simulink model "adcs_v16_integral_light_sun_sgp_igrf_power_7May2012"  (Simulink 7.5)
settings: Solver=ode1  StartTime=0.0  StopTime=120000  FixedStep=s_SIM_STEP_SIZE  RelTol=1e-3
values from neighbouring files (symbols this model uses):
  A = ((T_SIDE + .29)*1e-3)^2    [constants_v13.m]    (also in constants_v15.m; constants_v15_Pow.m; constants_v15_Pow_ss_error.m; constants_v16_integral_kartavya.m)
  Area_SP_S1 = 4*11*0.02025*0.04025    (= 0.03586275)    [constants_v15_Pow.m]    (also in constants_v15_Pow_ss_error.m; constants_v16_integral_light_sun_sgp_igrf_power_13Dec2011.m)
  Area_SP_S2 = 4*11*0.02025*0.04025    (= 0.03586275)    [constants_v15_Pow.m]    (also in constants_v15_Pow_ss_error.m; constants_v16_integral_light_sun_sgp_igrf_power_13Dec2011.m)
  Area_SP_S3 = 0.0    (= 0)    [constants_v15_Pow.m]    (also in constants_v15_Pow_ss_error.m; constants_v16_integral_light_sun_sgp_igrf_power_13Dec2011.m)
  Area_SP_S4 = 4*11*0.02025*0.04025    (= 0.03586275)    [constants_v15_Pow.m]    (also in constants_v15_Pow_ss_error.m; constants_v16_integral_light_sun_sgp_igrf_power_13Dec2011.m)
  Area_SP_S5 = 0.0    (= 0)    [constants_v15_Pow.m]    (also in constants_v15_Pow_ss_error.m; constants_v16_integral_light_sun_sgp_igrf_power_13Dec2011.m)
  Area_SP_S6 = 3*11*0.02025*0.04025    (= 0.0268970625)    [constants_v15_Pow.m]    (also in constants_v15_Pow_ss_error.m; constants_v16_integral_light_sun_sgp_igrf_power_13Dec2011.m)
  Ca_Solar_Drag = 1.4    [constants_v13.m]    (also in constants_v15.m; constants_v15_Pow.m; constants_v15_Pow_ss_error.m; constants_v16_integral_kartavya.m)
  Cd = 2.2    [constants_v13.m]    (also in constants_v15.m; constants_v15_Pow.m; constants_v15_Pow_ss_error.m; constants_v16_integral_kartavya.m)
  check_time = 60000    [constants_v13.m]    (also in constants_v15.m = 10000; constants_v15_Pow.m = 10000; constants_v15_Pow_ss_error.m = 10000; constants_v16_integral_kartavya.m = 10000)
  efficiany_solar_cell = 0.16    [constants_v15_Pow.m]    (also in constants_v15_Pow_ss_error.m; constants_v16_integral_light_sun_sgp_igrf_power_13Dec2011.m)
  equinox = datenum('21-Mar-2010 12:0:0')    [constants_v13.m]    (also in constants_v15.m; constants_v15_Pow.m; constants_v15_Pow_ss_error.m; constants_v16_integral_kartavya.m)
  I_MAX = 0.5    [constants_v13.m]    (also in constants_v15.m; constants_v15_Pow.m; constants_v15_Pow_ss_error.m; constants_v16_integral_kartavya.m)
  I_TORQUER = 3.6 / 7.31    (= 0.492476060192)    [constants_v13.m]    (also in constants_v15.m; constants_v15_Pow.m; constants_v15_Pow_ss_error.m; constants_v16_integral_kartavya.m)
  Kd = 2* m_INERTIA / (s_numOrbits * T_ORBIT )    [constants_v13.m]    (also in constants_v15.m = m_INERTIA * (2 + delta)* zeta * w; constants_v15_Pow.m = m_INERTIA * (2 + delta)* zeta * w; constants_v15_Pow_ss_error.m = m_INERTIA * (2 + delta)* zeta * w; constants_v16_integral_kartavya.m = m_INERTIA * (2 + delta)* zeta * w)
  Kdetumb = K_det*eye(3)    [constants_v13.m]    (also in constants_v15.m; constants_v15_Pow.m; constants_v15_Pow_ss_error.m; constants_v16_integral_kartavya.m)
  Ki = m_INERTIA * delta * zeta * w^3    [constants_v15.m]    (also in constants_v15_Pow.m; constants_v15_Pow_ss_error.m; constants_v16_integral_kartavya.m; constants_v16_integral_light_sun_sgp_igrf_power_13Dec2011.m)
  Kp = m_INERTIA / (s_numOrbits * T_ORBIT * zeta)^2    [constants_v13.m]    (also in constants_v15.m = m_INERTIA * (w*w + 2*delta*zeta^2*w^2); constants_v15_Pow.m = m_INERTIA * (w*w + 2*delta*zeta^2*w^2); constants_v15_Pow_ss_error.m = m_INERTIA * (w*w + 2*delta*zeta^2*w^2); constants_v16_integral_kartavya.m = m_INERTIA * (w*w + 2*delta*zeta^2*w^2))
  m_INERTIA = [Ixx Ixy Ixz; Ixy Iyy Iyz; Ixz Iyz Izz]    [constants_v13.m]    (also in constants_v15.m; constants_v15_Pow.m = 1*[Ixx Ixy Ixz; Ixy Iyy Iyz; Ixz Iyz Izz]; constants_v15_Pow_ss_error.m = 1*[Ixx Ixy Ixz; Ixy Iyy Iyz; Ixz Iyz Izz]; constants_v16_integral_kartavya.m)
  mu = 6.673e-11*5.9742e24    (= 398658366000000)    [constants_v13.m]    (also in constants_v15.m; constants_v15_Pow.m; constants_v15_Pow_ss_error.m; constants_v16_integral_kartavya.m)
  N = 40    [constants_v13.m]    (also in constants_v15.m; constants_v15_Pow.m; constants_v15_Pow_ss_error.m; constants_v16_integral_kartavya.m)
  P_momentum_flux_from_the_sun = 4.4e-6    (= 4.4e-06)    [constants_v13.m]    (also in constants_v15.m; constants_v15_Pow.m; constants_v15_Pow_ss_error.m; constants_v16_integral_kartavya.m)
  q_BI0 = euler2qBI(roll0,pitch0,yaw0)    [constants_v13.m]    (also in constants_v15.m; constants_v15_Pow.m; constants_v15_Pow_ss_error.m; constants_v16_integral_kartavya.m)
  s_FRAME_SIZE = 2    [constants_v13.m]    (also in constants_v15.m; constants_v15_Pow.m; constants_v15_Pow_ss_error.m; constants_v16_integral_kartavya.m)
  s_m_MAX = 0.95    [constants_v13.m]    (also in constants_v15.m; constants_v15_Pow.m; constants_v15_Pow_ss_error.m; constants_v16_integral_kartavya.m)
  s_MAG_B = 2.5e-5    (= 2.5e-05)    [constants_v13.m]    (also in constants_v15.m; constants_v15_Pow.m; constants_v15_Pow_ss_error.m; constants_v16_integral_kartavya.m)
  s_MAGMETER_WEIGHT = .9    (= 0.9)    [constants_v13.m]    (also in constants_v15.m; constants_v15_Pow.m; constants_v15_Pow_ss_error.m; constants_v16_integral_kartavya.m)
  s_SIM_STEP_SIZE = 0.1    [constants_v13.m]    (also in constants_v15.m; constants_v15_Pow.m; constants_v15_Pow_ss_error.m; constants_v16_integral_kartavya.m)
  s_SS_ADC_gain = 5    [constants_v13.m]    (also in constants_v15.m; constants_v15_Pow.m; constants_v15_Pow_ss_error.m; constants_v16_integral_kartavya.m)
  s_SS_ADC_res = 2^12 - 1    (= 4095)    [constants_v13.m]    (also in constants_v15.m; constants_v15_Pow.m; constants_v15_Pow_ss_error.m; constants_v16_integral_kartavya.m)
  s_SS_MAX_ANGLE = 85    [constants_v13.m]    (also in constants_v15.m; constants_v15_Pow.m; constants_v15_Pow_ss_error.m; constants_v16_integral_kartavya.m)
  s_TAU_W = 60    [constants_v13.m]    (also in constants_v15.m; constants_v15_Pow.m; constants_v15_Pow_ss_error.m; constants_v16_integral_kartavya.m)
  s_x_MAGMETER_BIAS = 50e-9    (= 5e-08)    [constants_v13.m]    (also in constants_v15.m; constants_v15_Pow.m; constants_v15_Pow_ss_error.m; constants_v16_integral_kartavya.m)
  side = 0.26    [constants_v13.m]    (also in constants_v15.m; constants_v15_Pow.m; constants_v15_Pow_ss_error.m; constants_v16_integral_kartavya.m)
  Snum = 6    [constants_v13.m]    (also in constants_v15.m; constants_v15_Pow.m; constants_v15_Pow_ss_error.m; constants_v16_integral_kartavya.m)
  Solar_Constant = 1353    [constants_v15_Pow.m]    (also in constants_v15_Pow_ss_error.m; constants_v16_integral_light_sun_sgp_igrf_power_13Dec2011.m)
  today = datenum('18-Oct-2010 10:30:0')    [constants_v13.m]    (also in constants_v15.m; constants_v15_Pow.m; constants_v15_Pow_ss_error.m; constants_v16_integral_kartavya.m)
  tol_q4 = 0.7    [constants_v13.m]    (also in constants_v15.m = 0.85; constants_v15_Pow.m = 0.85; constants_v15_Pow_ss_error.m = 0.85; constants_v16_integral_kartavya.m = 0.85)
  tol_w = 4e-3    (= 0.004)    [constants_v13.m]    (also in constants_v15.m; constants_v15_Pow.m; constants_v15_Pow_ss_error.m; constants_v16_integral_kartavya.m)
  tolw_n2d = 10e-3    (= 0.01)    [constants_v15.m]    (also in constants_v15_Pow.m; constants_v15_Pow_ss_error.m; constants_v16_integral_kartavya.m; constants_v16_integral_light_sun_sgp_igrf_power_13Dec2011.m)
  Ts_display = 6    [constants_v13.m]    (also in constants_v15.m; constants_v15_Pow.m; constants_v15_Pow_ss_error.m; constants_v16_integral_kartavya.m)
  v_COM_to_COP_b = [.2; 1.75; .2]*1e-2    [constants_v13.m]    (also in constants_v15.m; constants_v15_Pow.m; constants_v15_Pow_ss_error.m; constants_v16_integral_kartavya.m)
  v_S1 = [1 0 0]    [constants_v13.m]    (also in constants_v15.m; constants_v15_Pow.m; constants_v15_Pow_ss_error.m; constants_v16_integral_kartavya.m)
  v_S2 = [-1 0 0]    [constants_v13.m]    (also in constants_v15.m; constants_v15_Pow.m; constants_v15_Pow_ss_error.m; constants_v16_integral_kartavya.m)
  v_S3 = [0 1 0]    [constants_v13.m]    (also in constants_v15.m; constants_v15_Pow.m; constants_v15_Pow_ss_error.m; constants_v16_integral_kartavya.m)
  v_S4 = [0 -1 0]    [constants_v13.m]    (also in constants_v15.m; constants_v15_Pow.m; constants_v15_Pow_ss_error.m; constants_v16_integral_kartavya.m)
  v_S5 = [0 0 1]    [constants_v13.m]    (also in constants_v15.m; constants_v15_Pow.m; constants_v15_Pow_ss_error.m; constants_v16_integral_kartavya.m)
  v_S6 = [0 0 -1]    [constants_v13.m]    (also in constants_v15.m; constants_v15_Pow.m; constants_v15_Pow_ss_error.m; constants_v16_integral_kartavya.m)
  v_x_MOUNTING_THETA_ZYX_BODY_TORQUER = [1; 1; 1]* pi/180    [constants_v13.m]    (also in constants_v15.m; constants_v15_Pow.m; constants_v15_Pow_ss_error.m; constants_v16_integral_kartavya.m)
  wx0 = 2*pi/180    (= 0.0349065850399)    [constants_v13.m]    (also in constants_v15.m = 0.00174532925199; constants_v15_Pow.m = 1.74532925199e-05; constants_v15_Pow_ss_error.m = 2.01533262693e-05; constants_v16_integral_kartavya.m = 0.0174532925199)
  wy0 = 1*pi/180    (= 0.0174532925199)    [constants_v13.m]    (also in constants_v15.m = 0.00174532925199; constants_v15_Pow.m = 1.74532925199e-05; constants_v15_Pow_ss_error.m = 2.01533262693e-05; constants_v16_integral_kartavya.m = 0)
  wz0 = -2*pi/180    (= -0.0349065850399)    [constants_v13.m]    (also in constants_v15.m = 0.00174532925199; constants_v15_Pow.m = 1.74532925199e-05; constants_v15_Pow_ss_error.m = 2.01533262693e-05; constants_v16_integral_kartavya.m = -0.00872664625997)
libraries: simulink x9, commnoisgen2 x7, aerolibutil x2
(part 2 of 2)

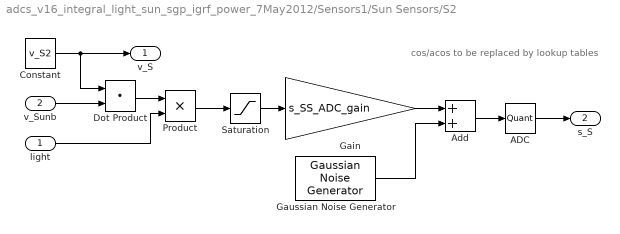
== system adcs_v16_integral_light_sun_sgp_igrf_power_7May2012/Sensors1/Sun Sensors/S2 ==
  note: cos/acos to be replaced by lookup tables
  light : Inport  OutDataType=sfix(16)  OutScaling=2^0
  v_Sunb : Inport  Port=2  OutDataType=sfix(16)  OutScaling=2^0
  ADC : Quantizer  QuantizationInterval=1/s_SS_ADC_res
  Add : Sum  OutDataType=sfix(16)  OutScaling=2^-10
  Constant : Constant  Value=v_S2  OutDataType=sfix(16)  OutScaling=2^0
  Dot Product : DotProduct  OutDataType=sfix(16)  OutScaling=2^-10  InputSameDT=on  OutDataTypeStr=Inherit: Inherit via internal rule
  Gain : Gain  Gain=s_SS_ADC_gain  ParameterDataType=sfix(16)  ParameterScaling=2^0  OutDataType=sfix(16)  OutScaling=2^0
  Gaussian Noise Generator : commnoisgen2/Gaussian Noise Generator  SystemSampleTime=-1  m=0  d=s_x_SUNSENSOR  s=41  Ts=s_SIM_STEP_SIZE  frameBased=off  sampPerFrame=1  orient=off  outDataType=double
  Product : Product  OutDataType=fixdt(1, 16)  OutScaling=2^0  RndMeth=Zero
  Saturation : Saturate  UpperLimit=inf  LowerLimit=0  OutDataType=sfix(16)  OutScaling=2^0
  v_S : Outport  OutDataType=sfix(16)  OutScaling=2^0
  s_S : Outport  Port=2  OutDataType=sfix(16)  OutScaling=2^0
  wires:
  ADC/1 -> s_S/1
  Add/1 -> ADC/1
  Gain/1 -> Add/1
  Gaussian Noise Generator/1 -> Add/2
  Constant/1 -> Dot Product/1, v_S/1
  Saturation/1 -> Gain/1
  v_Sunb/1 -> Dot Product/2
  Dot Product/1 -> Product/1
  Product/1 -> Saturation/1
  light/1 -> Product/2

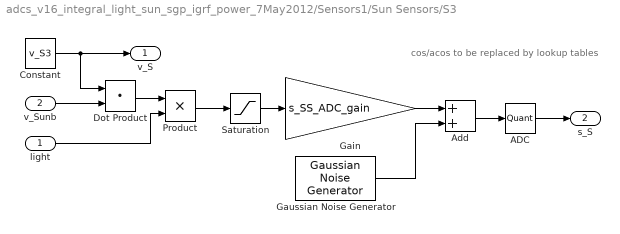
== system adcs_v16_integral_light_sun_sgp_igrf_power_7May2012/Sensors1/Sun Sensors/S3 ==
  note: cos/acos to be replaced by lookup tables
  light : Inport  OutDataType=sfix(16)  OutScaling=2^0
  v_Sunb : Inport  Port=2  OutDataType=sfix(16)  OutScaling=2^0
  ADC : Quantizer  QuantizationInterval=1/s_SS_ADC_res
  Add : Sum  OutDataType=sfix(16)  OutScaling=2^-10
  Constant : Constant  Value=v_S3  OutDataType=sfix(16)  OutScaling=2^0
  Dot Product : DotProduct  OutDataType=sfix(16)  OutScaling=2^-10  InputSameDT=on  OutDataTypeStr=Inherit: Inherit via internal rule
  Gain : Gain  Gain=s_SS_ADC_gain  ParameterDataType=sfix(16)  ParameterScaling=2^0  OutDataType=sfix(16)  OutScaling=2^0
  Gaussian Noise Generator : commnoisgen2/Gaussian Noise Generator  SystemSampleTime=-1  m=0  d=s_x_SUNSENSOR  s=41  Ts=s_SIM_STEP_SIZE  frameBased=off  sampPerFrame=1  orient=off  outDataType=double
  Product : Product  OutDataType=fixdt(1, 16)  OutScaling=2^0  RndMeth=Zero
  Saturation : Saturate  UpperLimit=inf  LowerLimit=0  OutDataType=sfix(16)  OutScaling=2^0
  v_S : Outport  OutDataType=sfix(16)  OutScaling=2^0
  s_S : Outport  Port=2  OutDataType=sfix(16)  OutScaling=2^0
  wires:
  light/1 -> Product/2
  Product/1 -> Saturation/1
  Dot Product/1 -> Product/1
  v_Sunb/1 -> Dot Product/2
  Saturation/1 -> Gain/1
  Constant/1 -> v_S/1, Dot Product/1
  Gaussian Noise Generator/1 -> Add/2
  Gain/1 -> Add/1
  Add/1 -> ADC/1
  ADC/1 -> s_S/1

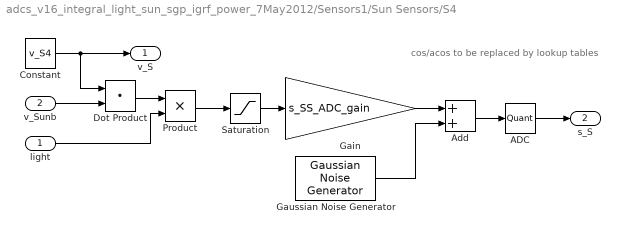
== system adcs_v16_integral_light_sun_sgp_igrf_power_7May2012/Sensors1/Sun Sensors/S4 ==
  note: cos/acos to be replaced by lookup tables
  light : Inport  OutDataType=sfix(16)  OutScaling=2^0
  v_Sunb : Inport  Port=2  OutDataType=sfix(16)  OutScaling=2^0
  ADC : Quantizer  QuantizationInterval=1/s_SS_ADC_res
  Add : Sum  OutDataType=sfix(16)  OutScaling=2^-10
  Constant : Constant  Value=v_S4  OutDataType=sfix(16)  OutScaling=2^0
  Dot Product : DotProduct  OutDataType=sfix(16)  OutScaling=2^-10  InputSameDT=on  OutDataTypeStr=Inherit: Inherit via internal rule
  Gain : Gain  Gain=s_SS_ADC_gain  ParameterDataType=sfix(16)  ParameterScaling=2^0  OutDataType=sfix(16)  OutScaling=2^0
  Gaussian Noise Generator : commnoisgen2/Gaussian Noise Generator  SystemSampleTime=-1  m=0  d=s_x_SUNSENSOR  s=41  Ts=s_SIM_STEP_SIZE  frameBased=off  sampPerFrame=1  orient=off  outDataType=double
  Product : Product  OutDataType=fixdt(1, 16)  OutScaling=2^0  RndMeth=Zero
  Saturation : Saturate  UpperLimit=inf  LowerLimit=0  OutDataType=sfix(16)  OutScaling=2^0
  v_S : Outport  OutDataType=sfix(16)  OutScaling=2^0
  s_S : Outport  Port=2  OutDataType=sfix(16)  OutScaling=2^0
  wires:
  ADC/1 -> s_S/1
  Add/1 -> ADC/1
  Gain/1 -> Add/1
  Gaussian Noise Generator/1 -> Add/2
  Constant/1 -> Dot Product/1, v_S/1
  Saturation/1 -> Gain/1
  v_Sunb/1 -> Dot Product/2
  Dot Product/1 -> Product/1
  Product/1 -> Saturation/1
  light/1 -> Product/2

== system adcs_v16_integral_light_sun_sgp_igrf_power_7May2012/Sensors1/Sun Sensors/S5 ==
  note: cos/acos to be replaced by lookup tables
  light : Inport  OutDataType=sfix(16)  OutScaling=2^0
  v_Sunb : Inport  Port=2  OutDataType=sfix(16)  OutScaling=2^0
  ADC : Quantizer  QuantizationInterval=1/s_SS_ADC_res
  Add : Sum  OutDataType=sfix(16)  OutScaling=2^-10
  Constant : Constant  Value=v_S5  OutDataType=sfix(16)  OutScaling=2^0
  Dot Product : DotProduct  OutDataType=sfix(16)  OutScaling=2^-10  InputSameDT=on  OutDataTypeStr=Inherit: Inherit via internal rule
  Gain : Gain  Gain=s_SS_ADC_gain  ParameterDataType=sfix(16)  ParameterScaling=2^0  OutDataType=sfix(16)  OutScaling=2^0
  Gaussian Noise Generator : commnoisgen2/Gaussian Noise Generator  SystemSampleTime=-1  m=0  d=s_x_SUNSENSOR  s=41  Ts=s_SIM_STEP_SIZE  frameBased=off  sampPerFrame=1  orient=off  outDataType=double
  Product : Product  OutDataType=fixdt(1, 16)  OutScaling=2^0  RndMeth=Zero
  Saturation : Saturate  UpperLimit=inf  LowerLimit=0  OutDataType=sfix(16)  OutScaling=2^0
  v_S : Outport  OutDataType=sfix(16)  OutScaling=2^0
  s_S : Outport  Port=2  OutDataType=sfix(16)  OutScaling=2^0
  wires:
  light/1 -> Product/2
  Product/1 -> Saturation/1
  Dot Product/1 -> Product/1
  v_Sunb/1 -> Dot Product/2
  Saturation/1 -> Gain/1
  Constant/1 -> v_S/1, Dot Product/1
  Gaussian Noise Generator/1 -> Add/2
  Gain/1 -> Add/1
  Add/1 -> ADC/1
  ADC/1 -> s_S/1

== system adcs_v16_integral_light_sun_sgp_igrf_power_7May2012/Sensors1/Sun Sensors/S6 ==
  note: cos/acos to be replaced by lookup tables
  light : Inport  OutDataType=sfix(16)  OutScaling=2^0
  v_Sunb : Inport  Port=2  OutDataType=sfix(16)  OutScaling=2^0
  ADC : Quantizer  QuantizationInterval=1/s_SS_ADC_res
  Add : Sum  OutDataType=sfix(16)  OutScaling=2^-10
  Constant : Constant  Value=v_S6  OutDataType=sfix(16)  OutScaling=2^0
  Dot Product : DotProduct  OutDataType=sfix(16)  OutScaling=2^-10  InputSameDT=on  OutDataTypeStr=Inherit: Inherit via internal rule
  Gain : Gain  Gain=s_SS_ADC_gain  ParameterDataType=sfix(16)  ParameterScaling=2^0  OutDataType=sfix(16)  OutScaling=2^0
  Gaussian Noise Generator : commnoisgen2/Gaussian Noise Generator  SystemSampleTime=-1  m=0  d=s_x_SUNSENSOR  s=41  Ts=s_SIM_STEP_SIZE  frameBased=off  sampPerFrame=1  orient=off  outDataType=double
  Product : Product  OutDataType=fixdt(1, 16)  OutScaling=2^0  RndMeth=Zero
  Saturation : Saturate  UpperLimit=inf  LowerLimit=0  OutDataType=sfix(16)  OutScaling=2^0
  v_S : Outport  OutDataType=sfix(16)  OutScaling=2^0
  s_S : Outport  Port=2  OutDataType=sfix(16)  OutScaling=2^0
  wires:
  ADC/1 -> s_S/1
  Add/1 -> ADC/1
  Gain/1 -> Add/1
  Gaussian Noise Generator/1 -> Add/2
  Constant/1 -> Dot Product/1, v_S/1
  Saturation/1 -> Gain/1
  v_Sunb/1 -> Dot Product/2
  Dot Product/1 -> Product/1
  Product/1 -> Saturation/1
  light/1 -> Product/2

== matlab function Torquer/Embedded MATLAB Function4 ==
  data: euler input double; DCM output double
function DCM  = f(euler)
% This block supports the Embedded MATLAB subset.
% See the help menu for details. 

roll = euler(1);
pitch = euler(2);
yaw = euler(3);

rot_x = [  1         0           0;...
             0         cos(roll)  sin(roll);...
             0        -sin(roll)  cos(roll)];
         
rot_y = [cos(pitch)   0       -sin(pitch);...
            0           1        0;...
           sin(pitch)   0        cos(pitch)];
       
rot_z = [ cos(yaw) sin(yaw) 0;...
           -sin(yaw) cos(yaw) 0;...
            0        0            1];
         
DCM  = rot_z *  rot_y *  rot_x;

== matlab function Embedded MATLAB Function ==
  data: x input double; u input double; xdot output double; m_INERTIA parameter double
function xdot = fcn(x, u, m_INERTIA)
% This block supports the Embedded MATLAB subset.
% See the help menu for details. 

q = x(1:4);
w = x(5:7);

W = ...
    [ 0 w(3) -w(2) w(1);
      -w(3) 0 w(1) w(2);
      w(2) -w(1) 0 w(3);
      -w(1) -w(2) -w(3) 0];
  
  qdot = 0.5 * W * q;
  wdot = inv(m_INERTIA)*( u - cross( w, m_INERTIA*w ) );
  
  xdot = [qdot; wdot];

== matlab function I -> B/L_Inertial ==
  data: x input double; v_B output double; v_I input double
function v_B = fcn(x, v_I)
% This block supports the Embedded MATLAB subset.
% See the help menu for details. 

q = x(1:4);

q0 = q(4); q1 = q(1); q2 = q(2); q3 = q(3);

TBI = [ q0^2 + q1^2 - q2^2 - q3^2,         2*q0*q3 + 2*q1*q2,         2*q1*q3 - 2*q0*q2;
           2*q1*q2 - 2*q0*q3, q0^2 - q1^2 + q2^2 - q3^2,         2*q0*q1 + 2*q2*q3;
           2*q0*q2 + 2*q1*q3,         2*q2*q3 - 2*q0*q1, q0^2 - q1^2 - q2^2 + q3^2];

v_B =  TBI*v_I;

== matlab function q -> w/Subsystem6/(1-L) + L/z ==
  data: a input double; y output double; b input double
function y = fcn(a,b)
%#eml

c = 1-a;

y = c+b;
if y>1
    y=1;
end

== matlab function q-normalise ==
  data: x input double; xN output double
function xN  = fcn(x)
% This block gives DCM for converting from ECI to ORBIT frames
% inputs: state vector in ECI
% output: DCM

q = x(1:4);
q = q/sqrt(dot(q,q));
xN = [q; x(5:7)];

== matlab function External Torques/Subsystem/Solar_drag ==
  data: v_Sun_b input double; solar_drag output double; Ca_Solar_Drag parameter double; P_momentum_flux_from_the_sun parameter double; light input double; side parameter double
function solar_drag = fcn(v_Sun_b,Ca_Solar_Drag,P_momentum_flux_from_the_sun,light, side)
% This block supports the Embedded MATLAB subset.
% See the help menu for details. 

% dot product of area vector and sun vector
if (norm(v_Sun_b) == 0)
    u = [1;0;0];
else
    u = v_Sun_b / norm(v_Sun_b);
end

y = 0 ;
a = side;
a = a*a; %Area of satellite
b =  zeros(3,6);
b(:,1) = a*[1;0;0];
b(:,2) = a*[0;1;0];
b(:,3) = a*[0;0;1];
b(:,4) = a*[-1;0;0];
b(:,5) = a*[0;-1;0];
b(:,6) = a*[0;0;-1];

x = 0;
for i=1:6
     x = dot(b(:,i),u);
    if(x>0)
            y = y+x;
    end
end
Ap = y;

solar_drag = -Ap * Ca_Solar_Drag * P_momentum_flux_from_the_sun * u * light;

== matlab function External Torques/L_Inertial ==
  data: x input double; tau output double; v_Si input double; mu parameter double; m_INERTIA parameter double
function tau = fcn(x, v_Si, mu, m_INERTIA)
% This block supports the Embedded MATLAB subset.
% See the help menu for details. 

q = x(1:4);

q0 = q(4); q1 = q(1); q2 = q(2); q3 = q(3);

TBI = [ q0^2 + q1^2 - q2^2 - q3^2,         2*q0*q3 + 2*q1*q2,         2*q1*q3 - 2*q0*q2;
           2*q1*q2 - 2*q0*q3, q0^2 - q1^2 + q2^2 - q3^2,         2*q0*q1 + 2*q2*q3;
           2*q0*q2 + 2*q1*q3,         2*q2*q3 - 2*q0*q1, q0^2 - q1^2 - q2^2 + q3^2];

r_I = v_Si(1:3);
r_B =  TBI*r_I;

R = sqrt(dot(r_B, r_B));
tau = 3*mu * cross( r_B, m_INERTIA*r_B) / R^5;

== matlab function Control Law/q->w ==
  data: B output double; B_l input double; B_k input double; dB output double; s_FRAME_SIZE parameter double
function [B, dB] = fcn(B_l, B_k, s_FRAME_SIZE)
% This block supports the Embedded MATLAB subset.
% See the help menu for details. 

dB = (B_l - B_k)/s_FRAME_SIZE;
B = (B_l + B_k)/2;

== matlab function QuEST ==
  data: v_Bb_m input double; m_SUN input double; q_BO_est output double; v_Bo_c input double; v_So_c input double; s_SS_ADC_gain parameter double; Snum parameter double; light_est output double; s_MAGMETER_WEIGHT parameter double; s_SS_MAX_ANGLE parameter double; v_Sun1 output double
function [q_BO_est, light_est, v_Sun1] = QuEST(v_Bb_m,m_SUN,v_Bo_c,v_So_c, s_SS_ADC_gain, Snum, s_MAGMETER_WEIGHT, s_SS_MAX_ANGLE)

    % Help
    % q_triad = Estimated quaternion
    % b1,b2 = the 2 measurement vectors in body frames
    % r1,r2 = the 2 measurement vectors in reference frames (orbit/inertial; orbit used)
    % b1 is the measurement with very high accurace as compared to b2
    % I am not sure how r1 and r2 will be determined
    % a1 and a2 are Relative weights of b1 and b2


%%%%% calculate v_Sb_m from m_SUN %%%%
t_S = ones(1,Snum)*cos(s_SS_MAX_ANGLE *pi/180);
m_SUN(4,:) = 1.0*(m_SUN(5,:)>t_S);     % set flags from measured voltages

values = m_SUN(5,:);

n_SS = 0;
for i=1:Snum
    if values(i) < 0.5*s_SS_ADC_gain
        n_SS = n_SS + 1;
    end
end

if (n_SS == Snum) 
    light = 0;
else
    light = 1;
end

light_est = light;
%v_Sun1 = [1;0;0];

if (light == 1)    
    
    %%% CALCULATE SUN VECTOR %%%
    
    ssvectors = zeros(3); ssvalues = zeros(3,1); ssflags = zeros(3,1);
     % flags = m_SUN(4,:)';
%     for i=1:3
%         [~, index] = sort(m_SUN(5,:));  % sort values in ascending order
%         z = index(Snum);
%         ssvectors(i,1:3) = m_SUN(1:3,z)';
%         ssflags(i) = m_SUN(4,z);
%         ssvalues(i) = m_SUN(5,z);
%         m_SUN(5,z) = -100 ;
%         for j= 1:Snum
%             if( norm(ssvectors(i,1:3)+m_SUN(1:3,j)') == 0 )
%                 m_SUN(5,j) = -100;
%             end
%         end
%     end
    
    [~, index] = sort(m_SUN(5,:));  % sort values in ascending order
    z = index(Snum); p = 0; % first vector
    ssvectors(1,1:3) = m_SUN(1:3,z)';
    ssvalues(1) = m_SUN(5,z);
    p = p+1;
    
    z = index(Snum-p);  % second vector
    while norm(m_SUN(1:3,z)' + ssvectors(1,1:3)) == 0
        p = p+1;
        z = index(Snum - p);
    end
    ssvectors(2,1:3) = m_SUN(1:3,z)';
    ssvalues(2) = m_SUN(5,z);
    p = p+1;
    
    z = index(Snum-p);  % 3rd vector
    while (norm(m_SUN(1:3,z)' + ssvectors(1,1:3)) == 0) || (norm(m_SUN(1:3,z)' + ssvectors(2,1:3)) == 0)
        p = p+1;
        z = index(Snum - p);
    end
    ssvectors(3,1:3) = m_SUN(1:3,z)';
    ssvalues(3) = m_SUN(5,z);
%     p = p+1;
    
    % v_Sun1 = inv(ssvectors)*ssvalues;
    v_Sun1 = ssvectors\ssvalues;
    v_Sun1 = v_Sun1/sqrt(dot(v_Sun1, v_Sun1));
    v_Sb_m = v_Sun1/sqrt(dot(v_Sun1, v_Sun1));
    
    %%%% start TRIAD %%%%

    b1 = v_Bb_m;
    b2 = v_Sb_m;
    r1 = v_Bo_c;
    r2 = v_So_c;

    a1 = s_MAGMETER_WEIGHT;
    a2 = 1-a1;

    %b3
    b3 = cross(b1,b2);
    b3 = b3/norm(b3) ;
    %r3
    r3 = cross(r1,r2);
    r3 = r3/norm(r3) ;

    %mu
    mu = ( 1 + dot(b3,r3) ) * ( a1*dot(b1,r1) + a2*dot(b2,r2) ) ;
    mu =  mu + dot( cross(b3,r3) , ( a1*cross(b1,r1) + a2*cross(b2,r2) ) ) ;

    %nu
    nu = dot( ( b3 + r3 ) , ( a1*cross(b1,r1) + a2*cross(b2,r2) )  ) ;

    %rho
    rho = sqrt( mu*mu + nu*nu );

    %q
    if( mu > 0)
        k_q_triad = (1/( 2*sqrt( rho*(rho+mu)*( 1 + dot(b3,r3) ) ) ) );
        v_q_triad = ( rho + mu )*( cross(b3,r3) ) + nu*(b3 + r3) ;
        s_q_triad = ( rho + mu )* ( 1 + dot(b3,r3) ) ;
        q_triad = [v_q_triad ; s_q_triad];
        q_triad = k_q_triad * q_triad ;
    else
        k_q_triad = (1/( 2*sqrt( rho*(rho-mu)*( 1 + dot(b3,r3) ) ) ) );
        v_q_triad = ( nu )*( cross(b3,r3) ) + ( rho - mu )*(b3 + r3) ;
        s_q_triad = ( nu )* ( 1 + dot(b3,r3) ) ;
        q_triad = [v_q_triad ; s_q_triad];
        q_triad = k_q_triad * q_triad ;    
    end

    q_triad = q_triad / sqrt(dot(q_triad,q_triad)) ;
    q_BO_est = q_triad;
else
    v_Sun1 = [1 ; 0 ; 0];
    q_BO_est = [0;0;0;1];
    flag_sum = 0;
end
end

== matlab function Satellite Computations I Propagators/m_TOI_NEW1 ==
  data: v_I input double; ECI input double; v_O output double
function v_O  = fcn(v_I, ECI)
% This block gives DCM for converting from ECI to ORBIT frames
% inputs: state vector in ECI
% output: DCM

r = ECI(1:3);   % position vector in ECI
v = ECI(4:6);   % velocity vector in ECI

oy = cross(v,r);    % orbit frame x...
oy = oy/sqrt(dot(oy,oy));

oz = -r/sqrt(dot(r,r));

ox = cross(oy,oz);
ox = ox/sqrt(dot(ox,ox));

TOI = [ox oy oz]';

v_O = TOI*v_I;

== matlab function Control Law/Nominal ==
  data: ieu output double; ieu_prev input double; eu output double; m output double; light input double; w input double; m_N output double; v_B input double; Kp parameter double; Kd parameter double; Ki parameter double; q input double; s_FRAME_SIZE parameter double
function [ieu, eu, m, m_N] = fcn(ieu_prev, light, w, v_B, Kp, Kd, Ki, q, s_FRAME_SIZE)
% This block supports the Embedded MATLAB subset.
% See the help menu for details. 

Bnorm = sqrt(dot(v_B, v_B));

q = q/sqrt(dot(q,q));

qv = q(1:3);    % e*sin(t/2)
qs = q(4);      %   cos(t/2)

eu = 2*qv*qs;     % 2*e*sin(t/2)*cos(t/2) = e*sin(t)    % P variable
         
ieu = ieu_prev + eu*s_FRAME_SIZE;   % integral eu dt,   % I variable

m = (Kp*eu + Ki*ieu + Kd*w) / Bnorm^2;

m_N = cross( m, v_B ) * light;

== matlab function Subsystem1/f: I->B ==
  data: x input double; v_B output double; v_I input double
function v_B = fcn(x, v_I)
% This block supports the Embedded MATLAB subset.
% See the help menu for details. 

q = x(1:4);

q0 = q(4); q1 = q(1); q2 = q(2); q3 = q(3);

TBI = [ q0^2 + q1^2 - q2^2 - q3^2,         2*q0*q3 + 2*q1*q2,         2*q1*q3 - 2*q0*q2;
           2*q1*q2 - 2*q0*q3, q0^2 - q1^2 + q2^2 - q3^2,         2*q0*q1 + 2*q2*q3;
           2*q0*q2 + 2*q1*q3,         2*q2*q3 - 2*q0*q1, q0^2 - q1^2 - q2^2 + q3^2];

v_B =  TBI*v_I;
v_B = v_B/sqrt(dot(v_B,v_B));

== matlab function External Torques/Aerodynamic Torque/aero torque ==
  data: v_B input double; u_aero output double; side parameter double; Cd parameter double; v_COM_to_COP_b parameter double
function u_aero = fcn( v_B,side, Cd, v_COM_to_COP_b)

% x = 1;
% z = x*1;
% y = z*u;

% This block supports an embeddable subset of the MATLAB language.
% See the help menu for details. 
% dot product of area vector and velocity vector
rho   = 1e-10;
vnorm = sqrt(dot(v_B,v_B));
v_unit = v_B / vnorm;

y = 0 ;
a = side;
a = a*a; %Area of satellite
b =  zeros(3,6);
b(:,1) = a*[1;0;0];
b(:,2) = a*[0;1;0];
b(:,3) = a*[0;0;1];
b(:,4) = a*[-1;0;0];
b(:,5) = a*[0;-1;0];
b(:,6) = a*[0;0;-1];

for i=1:6
     x = dot(b(:,i),v_unit);
    if(x>0)
            y = y+x;
    end
end
Ap = y; % total exposed area

F_aero = -0.5 * Cd * rho * Ap * vnorm^2 * v_unit;

u_aero = cross(v_COM_to_COP_b, F_aero);

== matlab function Power D0D/Watts x time/Embedded MATLAB Function ==
  data: Latitude input double; Longitude input double; Downlink_power output double; flag_downlink output double; flag_france output double; flag_india output double
function [Downlink_power, flag_downlink,flag_france,flag_india]  = fcn(Latitude, Longitude)
%#eml
phi = 10;
flag_france = 0;
flag_india = 0;
if (Latitude - 22.5833)^2 + cos(Latitude*pi/180)*(Longitude - 82.7666)^2 < (15 + phi)^2
    flag_downlink = 1;
    flag_india = 1;
elseif (Latitude - 48.8)^2 + cos(Latitude*pi/180)*(Longitude - 2.33)^2 < phi^2
    flag_downlink = 1;
    flag_france = 1;
else
    flag_downlink = 0;
end

Downlink_power = flag_downlink*2.6; %W
    
% 
% y = u;

== matlab function External Torques/Aerodynamic Torque/v_I to v_B ==
  data: v_I input double; x input double; v_B output double
function v_B = fcn(v_I,x)
% This block supports the Embedded MATLAB subset.
% See the help menu for details. 

q = x(1:4);

q0 = q(4); q1 = q(1); q2 = q(2); q3 = q(3);

TBI = [ q0^2 + q1^2 - q2^2 - q3^2,         2*q0*q3 + 2*q1*q2,         2*q1*q3 - 2*q0*q2;
           2*q1*q2 - 2*q0*q3, q0^2 - q1^2 + q2^2 - q3^2,         2*q0*q1 + 2*q2*q3;
           2*q0*q2 + 2*q1*q3,         2*q2*q3 - 2*q0*q1, q0^2 - q1^2 - q2^2 + q3^2];

v_B =  TBI*v_I;

== matlab function Sensors1/Sun Sensors/Embedded MATLAB Function ==
  data: v_S1 input double; m_SUN output double; s_S1 input double; v_S2 input double; s_S2 input double; v_S3 input double; s_S3 input double; v_S4 input double; s_S4 input double; v_S5 input double; s_S5 input double; v_S6 input double; s_S6 input double; Snum parameter double; s_SS_MAX_ANGLE parameter double; values output double
function [m_SUN, values] = fcn(v_S1, s_S1, v_S2, s_S2, v_S3, s_S3, v_S4, s_S4, v_S5, s_S5, v_S6, s_S6, Snum, s_SS_MAX_ANGLE)

a = cos(s_SS_MAX_ANGLE *pi/180);
t_S = ones(1,6)*a;

m_SUNtot = [v_S1 v_S2 v_S3 v_S4 v_S5 v_S6 ; % SS vectors
               0    0    0    0    0    0 ; % flags
            s_S1 s_S2 s_S3 s_S4 s_S5 s_S6 ];% values
        
m_SUNtot(4,:) = 1.0*(m_SUNtot(5,:)>t_S);

m_SUN = m_SUNtot(:, 1:Snum);
values = m_SUN(5,:)';

== matlab function Control Law/Detumbling ==
  data: v_B input double; Bdot input double; Kdetumb parameter double; m_D output double; s_MAG_B parameter double
function m_D = fcn(v_B, Bdot, Kdetumb, s_MAG_B)
% This block supports the Embedded MATLAB subset.
% See the help menu for details. 

Bnorm = sqrt(dot(v_B, v_B));
m_D = -Kdetumb * Bdot * (s_MAG_B / Bnorm);

== matlab function Control Law/Switching Algorithm/gate pulse ==
  data: N_prev input double; w input double; q input double; tol_w parameter double; tolw_n2d parameter double; N output double; P output double; tol_q4 parameter double; t input double; check_time parameter double; light_flag input double; w_ctrl input double; t_now output double; t_now_prev input double
function [N,P,t_now] = fcn( N_prev, w, q, tol_w, tolw_n2d, tol_q4, t,check_time, light_flag, w_ctrl,t_now_prev)

modw = sqrt(dot(w, w));
switch_d2n = (modw < tol_w) && (light_flag*w_ctrl ==1);
switch_n2d = (modw > tolw_n2d);

% condition check - DEBUG purpose
P = [1.0*(abs(q(4)) > tol_q4) + 0.1; 
     1.0*(modw < tol_w);
     1.0*(light_flag*w_ctrl == 1) + 0.3];
%%%%%%%%%%%

N = N_prev;
t_now = t_now_prev;

if t < 2000
    N = 0;
    t_now = 0;
end

if ((switch_d2n == 1) && (N_prev == 0))
    N = 1;
    t_now = t;
end

if ((switch_n2d == 1) && (N_prev == 1) && (t > t_now_prev + check_time) )
    N = 0;
    t_now = t;
end

== matlab function Satellite Computations I Propagators/m_TOI_NEW ==
  data: ECI input double; v_O output double; v_I input double
function v_O  = fcn(ECI, v_I)
% This block gives DCM for converting from ECI to ORBIT frames
% inputs: state vector in ECI
% output: DCM

r = ECI(1:3);   % position vector in ECI
v = ECI(4:6);   % velocity vector in ECI

oy = cross(v,r);    % orbit frame x...
oy = oy/sqrt(dot(oy,oy));

oz = -r/sqrt(dot(r,r));

ox = cross(oy,oz);
ox = ox/sqrt(dot(ox,ox));

TOI = [ox oy oz]';

v_O = TOI*v_I;

== matlab function Power D0D/battery_DOD/Embedded MATLAB Function ==
  data: clk input double; Batt_cap output double; batt_cap input double; watts_time input double; VBat output double; flag_charge input double; Flag_charge output double; frac_Batt_cap output double; flag_discharge input double; Flag_discharge output double; s_SIM_STEP_SIZE parameter double; vbat input double; current output double
function [Batt_cap, VBat, Flag_charge, frac_Batt_cap, Flag_discharge, current]= fcn(clk, batt_cap, watts_time, flag_charge, flag_discharge, s_SIM_STEP_SIZE, vbat)
%#eml
% E0 = 4.0085; R = 0.016818; K = 0.0094937; A = 0.31425; B = 27.7554;
% alp = 0.001; bet = 0.005;
% for i=1:1:sizex(2)
%     y(i) = 0.45*exp(-alp*x(i)) + 3.75 - exp(bet*(x(i)-2200)); 
% end
% current = -2.2; %Amps  graph internal resistant = 80mohms
internal_resistance = 0.08; %ohms

if (clk<0.15)
    Batt_cap = 2000; % x 6 batteries (reduced battery capacity by 360 mAh assuming 1 mA consumption)
    current = 0; %Amps
    VBat = isro_battery( (2200-Batt_cap), current, internal_resistance );
    Flag_charge = 0;
    Flag_discharge = 0;
else
       
    if watts_time < 0
        current = watts_time/(s_SIM_STEP_SIZE*2*vbat);
        Batt_cap = batt_cap + watts_time/(3.6*6*vbat);
        VBat = isro_battery( (2200-Batt_cap) , current, internal_resistance );
    else
        if flag_charge == 1
            current = watts_time/(s_SIM_STEP_SIZE*2*vbat);
            Batt_cap = batt_cap + watts_time/(3.6*6*vbat);
            VBat = isro_battery( (2200-Batt_cap), current, internal_resistance );
        else
            current = 0;
            Batt_cap = batt_cap;
            VBat = isro_battery( (2200-Batt_cap), current, internal_resistance );
        end
    end
end

if VBat < 3.95;
    Flag_charge = 1;
else
    if VBat > 4.25;
        Flag_charge = -2;
    else
        Flag_charge = flag_charge;
    end
end
    
frac_Batt_cap = Batt_cap / 2199;

if VBat < 3.5
    Flag_discharge = 1;
else 
    Flag_discharge = 0;
end

== matlab function q -> w/q->w ==
  data: w_l output double; w_k input double; q_BI_l input double; q_BI_k input double; w output double; s_FRAME_SIZE parameter double; s_TAU_W parameter double
function [w_l,w] = fcn(w_k, q_BI_l, q_BI_k, s_FRAME_SIZE, s_TAU_W)
% This block supports the Embedded MATLAB subset.
% See the help menu for details. 
dq = (q_BI_l - q_BI_k)/s_FRAME_SIZE;
q = (q_BI_l + q_BI_k)/2;

de = dq(1:3);
e = q(1:3);
n = q(4);

ex = [0    -e(3)  e(2);
      e(3)     0 -e(1);
     -e(2)  e(1)    0];

w = 2*(n*n*eye(3) - n*ex + e*e')*de/n;

% filtering:

a = s_FRAME_SIZE/(s_FRAME_SIZE + s_TAU_W);
w_l = a*w + (1-a)*w_k;

== matlab function Power D0D/r_ECEF -> r_LLA ==
  data: r_ECEF input double; Latitutde output double; Longitude output double; Altitude output double
function [Latitutde, Longitude, Altitude] = fcn(r_ECEF)
%r_ECEF: ECEF position vector (in m)
%r_LLA: LLA postion vector (in rad, m)

radius_earth = 6371000;
r = norm(r_ECEF);
x = r_ECEF(1);
y = r_ECEF(2);
z = r_ECEF(3);

lat = asin(z/r);
long = atan2(y,x);
if (long < 0)
    long = long + 2*pi;
end
h = r - radius_earth;

Latitutde = lat*180/pi; %deg
Longitude = long*180/pi; %deg
Altitude  = h; %m
%r_LLA = [lat;long;h];

== matlab function Embedded MATLAB Function4 ==
  data: x input double; euler output double; v_Si input double; q_BO output double; w_BOB output double; modw output double; s_W_SAT parameter double; w_BIB output double
function [euler, q_BO, w_BOB, modw, w_BIB] = a(x,v_Si, s_W_SAT)
% This block supports the Embedded MATLAB subset.
% See the help menu for details. 

% ECI to TIO 
r = v_Si(1:3);   % position vector in ECI
v = v_Si(4:6);   % velocity vector in ECI

oy = cross(v,r);    % orbit frame x...
oy = oy/sqrt(dot(oy,oy));

oz = -r/sqrt(dot(r,r));

ox = cross(oy,oz);
ox = ox/sqrt(dot(ox,ox));

TIO = [ox oy oz];

% qIO from TIO
if (trace(TIO) == -1)
    if ( TIO(1,2) == 0 && TIO(1,3) ==0 )
        q_IO = [1; 0; 0; 0];
    elseif ( TIO(1,2) == 0 && TIO(2,3) ==0 )
        q_IO = [0; 1; 0; 0];
    elseif ( TIO(1,3) == 0 && TIO(2,3) ==0 )
        q_IO = [0; 0; 1; 0];
    else
        e1 = TIO(1,2)*TIO(1,3);
        e2 = TIO(1,2)*TIO(2,3);
        e3 = TIO(1,3)*TIO(2,3);
        norm = sqrt( e1*e1 + e2*e2 + e3*e3);
        q_IO = [e1; e2; e3; 0]/norm;
    end        
else
    q4 = 0.5*sqrt(1 + trace(TIO));
    q1 = -(TIO(3,2) - TIO(2,3)) / (4*q4);
    q2 = -(TIO(1,3) - TIO(3,1)) / (4*q4);
    q3 = -(TIO(2,1) - TIO(1,2)) / (4*q4);
    q_IO = [q1; q2; q3; q4];
end

q_BI = x(1:4);

% q_BO = q_BI*q_IO
q_BIx = ...
[ q_BI(4)  q_BI(3) -q_BI(2) q_BI(1);
 -q_BI(3)  q_BI(4)  q_BI(1) q_BI(2);
  q_BI(2) -q_BI(1)  q_BI(4) q_BI(3);
 -q_BI(1) -q_BI(2) -q_BI(3) q_BI(4)];

q_BO = q_BIx * q_IO;

euler =  (180/pi)*[atan2( 2*( q_BO(4)*q_BO(1)-q_BO(2)*q_BO(3) ),( 1 - 2*( q_BO(1)^2 + q_BO(2)^2 ) )  ) ;
              asin( 2*(q_BO(4)*q_BO(2)+q_BO(3)*q_BO(1)) );
             atan2( 2*( q_BO(4)*q_BO(3)-q_BO(1)*q_BO(2) ),( 1 - 2*( q_BO(2)^2 + q_BO(3)^2 ) )  ) ];
         
w_BIB = x(5:7);
w_OIO = [0; -s_W_SAT; 0];

q0 = q_BO(4); q1 = q_BO(1); q2 = q_BO(2); q3 = q_BO(3);

TBO = [ q0^2 + q1^2 - q2^2 - q3^2,         2*q0*q3 + 2*q1*q2,         2*q1*q3 - 2*q0*q2;
           2*q1*q2 - 2*q0*q3, q0^2 - q1^2 + q2^2 - q3^2,         2*q0*q1 + 2*q2*q3;
           2*q0*q2 + 2*q1*q3,         2*q2*q3 - 2*q0*q1, q0^2 - q1^2 - q2^2 + q3^2];
       
w_OIB = TBO*w_OIO;
w_BOB = w_BIB - w_OIB;

modw = sqrt(dot(w_BOB,w_BOB));

== matlab function Power D0D/r_ECI -> r_ECEF ==
  data: today parameter double; r_ECEF output double; equinox parameter double; r_I input double; t input double
function r_ECEF = fcn(today,equinox,r_I,t)
%u: position vector in ECI (in m)
%y: position vector in ECEF (in m)

stperut = 1.00273790935;    % siderial time = stperut * universal time
W_EARTH_ROT = 2*pi/86141;   % sidereal rotation angular velocity of earth, SI

ut_sec = (today - equinox)*24*60*60 + t; % universal time vector in sec
st_sec = stperut*ut_sec;    % sidereal time vector in sec

phi = st_sec*W_EARTH_ROT;            % sidereal time vector in rad

TEI = [ cos(phi) sin(phi) 0;
       -sin(phi) cos(phi) 0;
        0        0        1];

r_ECEF = TEI*r_I;

== matlab function Power D0D/Watts x time/Embedded MATLAB Function1 ==
  data: Vbat input double; pow input double; pow_drawn output double
function pow_drawn = fcn(Vbat,pow)
% This block supports the Embedded MATLAB subset.
% See the help menu for details. 

battery = 0;

if Vbat>3.0
    battery = 1;
else
    battery = 0;
end

if battery == 1
    pow_drawn = pow;
else
    pow_drawn = 0;
end
